simulink model "pid_controller1"  (R2014a)
settings: Solver=FixedStepDiscrete  StartTime=0.0  StopTime=10.0  FixedStep=Ts  RelTol=1e-3
values from neighbouring files (symbols this model uses):
  Fs = single(100)    [pid_controller1_ws.m]
  Kd = single(0.0081)    [pid_controller1_ws.m]
  Ki = single(0.387)    [pid_controller1_ws.m]
  Kp = single(1.53)    [pid_controller1_ws.m]
  Ts = double(0.01)    [pid_controller1_ws.m]
CloseFcn:
  | rtwprivate ssgencode ModelCloseRequest pid_controller
settings Model: BufferReuse=off  Creator=y_yama  LastModifiedBy=yoshi12
settings DataIOCC: SignalLoggingSaveFormat=ModelDataLogs
settings OptimizationCC: BlockReduction=off  InlineParams=on  OptimizeBlockIOStorage=off  BufferReuse=off  GlobalBufferReuse=off  ExpressionFolding=off  ExpressionDepthLimit=2147483647  LocalBlockOutputs=off  InitFltsAndDblsToZero=on  OptimizeModelRefInitCode=on  LifeSpan=1
settings DebuggingCC: SaveWithParameterizedLinksMsg=none  UnderspecifiedInitializationDetection=Classic  SignalResolutionControl=TryResolveAllWithWarning  MultiTaskDSMMsg=warning  MultiTaskCondExecSysMsg=none  FcnCallInpInsideContextMsg=UseLocalSettings  StateNameClashWarn=warning
settings HardwareCC: ProdIntDivRoundTo=Zero  ProdEndianess=LittleEndian  ProdHWDeviceType=Intel->x86/Pentium
settings RTWCC: SystemTargetFile=ert.tlc  GenCodeOnly=on  TemplateMakefile=ert_default_tmf  Description=Embedded Coder  GenerateReport=on  ProcessScript=ert_make_rtw_hook  IncludeHyperlinkInReport=on  LaunchReport=on  IncludeERTFirstTime=on  GenerateTraceInfo=on  GenerateTraceReport=on  GenerateTraceReportSl=on  GenerateTraceReportSf=on  GenerateTraceReportEml=on
settings CodeAppCC: IgnoreCustomStorageClasses=off  CustomSymbolStrType=$N$R$M  InternalIdentifier=Classic
settings ERTTargetCC: ParMdlRefBuildCompliant=on  CompOptLevelCompliant=on  ConcurrentExecutionCompliant=on  ERTFirstTimeCompliant=on  ModelStepFunctionPrototypeControlCompliant=on  CPPClassGenCompliant=on  ERTCustomFileTemplate=example_file_process.tlc

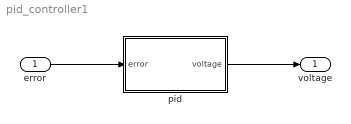
== system pid_controller1 ==
  error : Inport  OutDataTypeStr=single  PortDimensions=1  SampleTime=Ts
      settings: AttributesFormatString=<tsample = %<SampleTime>>
  pid : Subsystem
  voltage : Outport  OutDataTypeStr=single
  wires:
  pid/1(voltage) -> voltage/1
  error/1 -> pid/1(error)

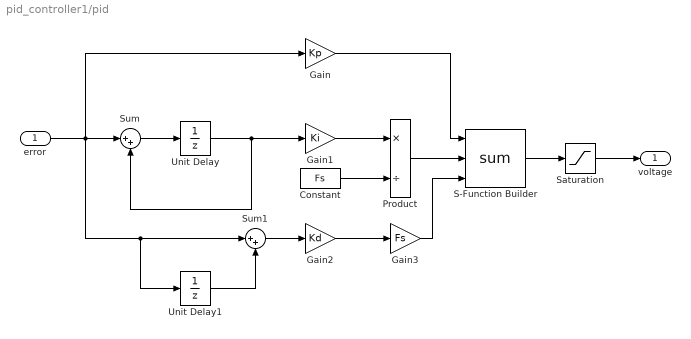
== system pid_controller1/pid ==
  error : Inport
  Constant : Constant  Value=Fs  SampleTime=Ts
  Gain : Gain  Gain=Kp  OutDataTypeStr=Inherit: Same as input
  Gain1 : Gain  Gain=Ki  OutDataTypeStr=Inherit: Same as input
  Gain2 : Gain  Gain=Kd  OutDataTypeStr=Inherit: Same as input
  Gain3 : Gain  Gain=Fs  OutDataTypeStr=Inherit: Same as input
  Product : Product  Inputs=*/  RndMeth=Zero  OutDataTypeStr=Inherit: Same as first input
  S-Function Builder : S-Function  InitFcn=try, set_param(gcb,'FunctionName','sum'), end  FunctionName=sum  SFunctionModules=sum_wrapper  EnableBusSupport=off  mask(S-Function Builder){}
      mask help: Simulink:masks:SFunctionBuilder_MD
      mask init:
      | val = [[.9  0.75 0.75 1 1 .9 .9 1]',[1 1 0.75 0.75 .9 .9 1 .9]'];try , sys = get_param(gcb,'SfunBuilderFcnName');if isempty(sys), sys = get_param(gcb,'FunctionName'); end,catch, sys = get_param(gcb,'FunctionName'); end
      settings: CopyFcn=set_param(gcbh,'LinkStatus','none')  PreSaveFcn=try, set_param(gcb,'FunctionName','sum'), end  OpenFcn=sfunctionwizard(gcbh)
      mask Display: plot(val(:,1),val(:,2)),disp(sys), port_label('input',1,'u0'), port_label('input',2,'u1'), port_label('input',3,'u2'), port_label('output',1,'y0')
  Saturation : Saturate  UpperLimit=5  LowerLimit=-5
      settings: AttributesFormatString=<limits = %<UpperLimit> / %<LowerLimit>>
  Sum : Sum  Inputs=|++
  Sum1 : Sum  Inputs=|++
  Unit Delay : UnitDelay  SampleTime=-1
      settings: AttributesFormatString=<identifer = %<StateIdentifier>>\n<initial = %<X0>>\n<tsample = %<SampleTime>>
  Unit Delay1 : UnitDelay  SampleTime=-1
      settings: AttributesFormatString=<identifer = %<StateIdentifier>>\n<initial = %<X0>>\n<tsample = %<SampleTime>>
  voltage : Outport
  wires:
  Unit Delay/1 -> Sum/2, Gain1/1
  Gain/1 -> S-Function Builder/1
  Unit Delay1/1 -> Sum1/2
  Sum1/1 -> Gain2/1
  S-Function Builder/1 -> Saturation/1
  Saturation/1 -> voltage/1
  Gain2/1 -> Gain3/1
  Gain1/1 -> Product/1
  Constant/1 -> Product/2
  Product/1 -> S-Function Builder/2
  Gain3/1 -> S-Function Builder/3
  error/1 -> Sum/1, Sum1/1, Unit Delay1/1, Gain/1
  Sum/1 -> Unit Delay/1
